simulink subsystem "ComputeDoA"  (R2021a)
settings: Solver=VariableStepAuto  StartTime=0.0  StopTime=10.0  RelTol=1e-3
settings Model: Creator=zurnmar  LastModifiedBy=zurnmar

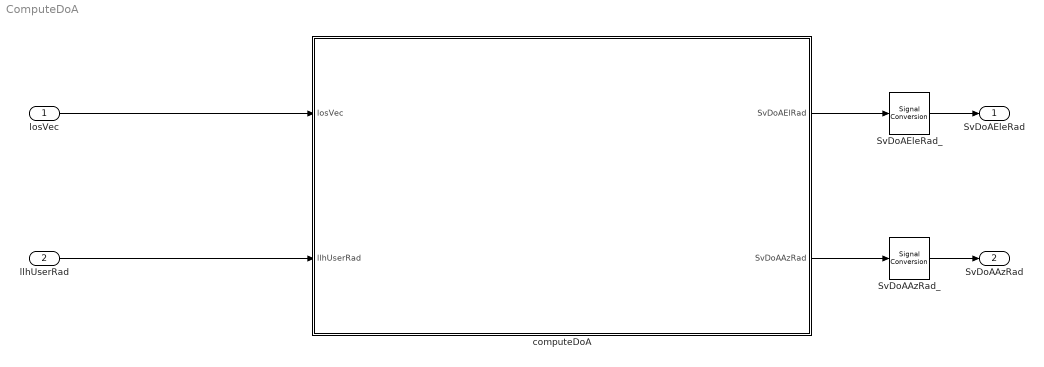
== system ComputeDoA ==
  losVec : Inport  PortDimensions=[3,1]
  llhUserRad : Inport  Port=2  PortDimensions=[3,1]
  SvDoAAzRad_ : SignalConversion  OverrideOpt=off
  SvDoAEleRad_ : SignalConversion  OverrideOpt=off
  computeDoA : MATLAB Function  TreatAsAtomicUnit=on
  SvDoAEleRad : Outport
  SvDoAAzRad : Outport  Port=2
  wires:
  computeDoA/1(SvDoAElRad) -> SvDoAEleRad_/1
  losVec/1 -> computeDoA/1(losVec)
  llhUserRad/1 -> computeDoA/2(llhUserRad)
  computeDoA/2(SvDoAAzRad) -> SvDoAAzRad_/1
  SvDoAEleRad_/1 -> SvDoAEleRad/1
  SvDoAAzRad_/1 -> SvDoAAzRad/1

== matlab function ComputeDoA/computeDoA ==
  data: losVec input; SvDoAElRad output; llhUserRad input; SvDoAAzRad output
function [SvDoAElRad,SvDoAAzRad] = computeDoA(losVec,llhUserRad)

SvDoAElRad=0;
SvDoAAzRad=0;
dV_rot=zeros(3,1);
phi = llhUserRad(1,1);
lam = llhUserRad(2,1);


sinphi = sin(phi);
cosphi = cos(phi);
sinlam = sin(lam);
coslam = cos(lam);
cosphicoslam = cosphi .* coslam;
cosphisinlam = cosphi .* sinlam;
sinphicoslam = sinphi .* coslam;
sinphisinlam = sinphi .* sinlam;


dV_rot = [-sinphicoslam -sinphisinlam cosphi ;...
    -sinlam        coslam       0;...
    cosphicoslam  cosphisinlam sinphi] * losVec;
SvDoAElRad  = ( 0.5 - atan2( sqrt(dV_rot(1)^2+dV_rot(2)^2), dV_rot(3)) / pi ) * pi;
SvDoa_azi_rad_1  = atan2(dV_rot(2),dV_rot(1));

if SvDoa_azi_rad_1<=0
    SvDoAAzRad = SvDoa_azi_rad_1 + 2*pi;
else
    SvDoAAzRad = SvDoa_azi_rad_1;
end


end
